simulink model "model_FS_PSH_IEEE39"  (R2020b)
settings: Solver=ode3  StartTime=0.0  StopTime=300  FixedStep=Ts  RelTol=1e-3
PostLoadFcn:
  | IEEE39BusLineLength;
  | vNomHV = 345E3;fNom=60;load('Dynamicload.mat');
InitFcn:
  | IEEE39BusLineLength;
  | vNomHV = 345E3;fNom=60;load('Dynamicload.mat');
values from neighbouring files (symbols this model uses):
  Rp = 0.05    [IEEE39BusLineLength.m]
  t_sw_off = 220    [MAIN_FS_PSH_IEEE39.m]    (also in MAIN_T_PSH_IEEE39.m; MAIN_VS_PSH.m = 45)
  t_sw_on = 130    [MAIN_FS_PSH_IEEE39.m]    (also in MAIN_T_PSH_IEEE39.m; MAIN_VS_PSH.m = 35)
  TL_10_11_len = 14    [IEEE39BusLineLength.m]
  TL_10_13_len = 14    [IEEE39BusLineLength.m]
  TL_13_14_len = 32    [IEEE39BusLineLength.m]
  TL_14_15_len = 70    [IEEE39BusLineLength.m]
  TL_15_16_len = 31.5    [IEEE39BusLineLength.m]
  TL_16_17_len = 26    [IEEE39BusLineLength.m]
  TL_16_19_len = 61    [IEEE39BusLineLength.m]
  TL_16_21_len = 46    [IEEE39BusLineLength.m]
  TL_16_24_len = 15    [IEEE39BusLineLength.m]
  TL_17_18_len = 26    [IEEE39BusLineLength.m]
  TL_17_27_len = 59    [IEEE39BusLineLength.m]
  TL_1_2_len = 134    [IEEE39BusLineLength.m]
  TL_1_39_len = 105    [IEEE39BusLineLength.m]
  TL_21_22_len = 47    [IEEE39BusLineLength.m]
  TL_22_23_len = 33    [IEEE39BusLineLength.m]
  TL_24_23_len = 88    [IEEE39BusLineLength.m]
  TL_25_26_len = 101    [IEEE39BusLineLength.m]
  TL_26_27_len = 46.5    [IEEE39BusLineLength.m]
  TL_26_28_len = 151    [IEEE39BusLineLength.m]
  TL_26_29_len = 200    [IEEE39BusLineLength.m]
  TL_28_29_len = 48    [IEEE39BusLineLength.m]
  TL_2_25_len = 28    [IEEE39BusLineLength.m]
  TL_2_2_len = 49    [IEEE39BusLineLength.m]
  TL_3_18_len = 42    [IEEE39BusLineLength.m]
  TL_3_4_len = 53    [IEEE39BusLineLength.m]
  TL_4_14_len = 33    [IEEE39BusLineLength.m]
  TL_4_5_len = 32.5    [IEEE39BusLineLength.m]
  TL_5_6_len = 14    [IEEE39BusLineLength.m]
  TL_5_8_len = 32    [IEEE39BusLineLength.m]
  TL_6_11_len = 26.5    [IEEE39BusLineLength.m]
  TL_6_7_len = 25.5    [IEEE39BusLineLength.m]
  TL_7_8_len = 15    [IEEE39BusLineLength.m]
  TL_8_9_len = 93    [IEEE39BusLineLength.m]
  TL_9_39_len = 136    [IEEE39BusLineLength.m]
  Ts = 25e-6    (= 2.5e-05)    [MAIN_FS_PSH_IEEE39.m]    (also in MAIN_T_PSH_IEEE39.m; MAIN_VS_PSH.m = 1e-07)
undefined symbols (not defined in the file or in its folder): D1, Delta, FS_PSH, load15, load16, load18, load20, load21, load23, load24, load25, load26, load27, load28, load29, load3, load39, load4, load7, load8
libraries: powerlib x216, sps_avr x10, powerlib_meascontrol x5, pid_lib x1
(part 1 of 8)
settings Model: ARTEMISmethode_block_infos=$$__separator__$$IEEE39bus_60Hz/ARTEMIS Guide$$__separator__$$  SimulationMode=accelerator  Creator=Admin  LastModifiedBy=mjimene
settings DataIOCC: LimitDataPoints=on  SaveFormat=Array  SignalLoggingSaveFormat=ModelDataLogs  SaveOutput=off  SignalLogging=off  DSMLogging=off  SaveTime=off
settings OptimizationCC: BlockReduction=off  OptimizeBlockIOStorage=off  BufferReuse=off  GlobalBufferReuse=off  ExpressionFolding=off  ExpressionDepthLimit=2147483647  LocalBlockOutputs=off  LifeSpan=inf
settings DebuggingCC: UnderspecifiedInitializationDetection=Classic  MergeDetectMultiDrivingBlocksExec=none  SolverPrmCheckMsg=warning  FcnCallInpInsideContextMsg=warning  UnconnectedInputMsg=none  UnconnectedOutputMsg=none  UnconnectedLineMsg=none  StateNameClashWarn=warning  SFUnexpectedBacktrackingDiag=warning  SFNoUnconditionalDefaultTransitionDiag=warning  SFExecutionAtInitializationDiag=none  ArithmeticOperatorsInVariantConditions=warning
settings HardwareCC: ProdBitPerPointer=32  ProdBitPerSizeT=32  ProdBitPerPtrDiffT=32  ProdLargestAtomicFloat=None  ProdIntDivRoundTo=Undefined  ProdEndianess=Unspecified  ProdWordSize=32  ProdHWDeviceType=32-bit Generic
settings ModelReferenceCC: PropagateSignalLabelsOutOfModel=off
settings SFSimCC: SimUseLocalCustomCode=off  CustomCodeUndefinedFunction=UseInterfaceOnly
settings RTWCC: RTWUseLocalCustomCode=off
settings CodeAppCC: StateflowObjectComments=on
settings GRTTargetCC: TargetLangStandard=C89/C90 (ANSI)  CombineOutputUpdateFcns=off  GRTInterface=on
settings ConfigComp: CovMetricSettings=dw  CovSaveCumulativeToWorkspaceVar=on  CovSaveSingleToWorkspaceVar=on  CovExternalEMLEnable=off
settings SimscapeCC: SimscapeNormalizeSystem=off

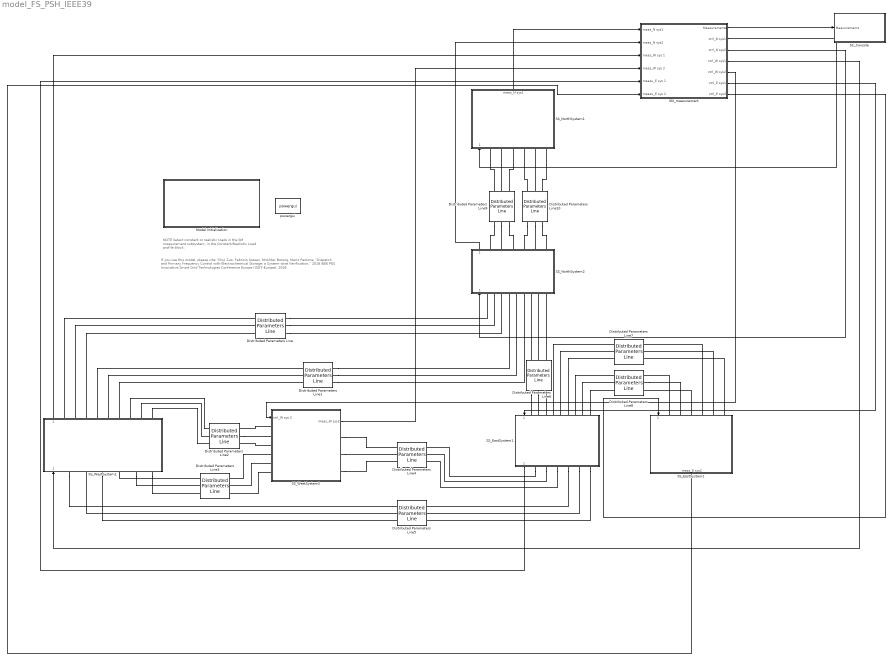
== system model_FS_PSH_IEEE39 ==
  note: If you use this model, please cite:
      | Yihui Zuo, Fabrizio Sossan, Mokhtar Bozorg, Mario Paolone,
      | “Dispatch and Primary Frequency Control with Electrochemical Storage: a System-wise Verification,”
      | 2018 IEEE PES Innovative Smart Grid Technologies Conference Europe (ISGT-Europe), 2018.
  note: NOTE
      | Select constant or realistic loads in the SM measurement
      | subsystem, in the Constant/Realistic Load profile block.
  Distributed Parameters Line : powerlib/Elements/Distributed Parameters Line  Phases=3  Length=TL_1_39_len  Frequency=fNom  Resistance=[1.19 4.76]/TL_1_39_len  Inductance="[0.079  0.237]/TL_1_39_len"  Capacitance=[1.67e-6 0.7599e-6]/TL_1_39_len  x1=[-0.000425 4.88875301437083e-09 0 0;-0.0004 4.8690649712249e-09 0 0;-0.000375 4.84894442957481e-09 175040.631407091 -214779.963387365;-0.00035 4.8283931766434e-09 177057.068450198 -213120.729509055;-0.000325 4.80741303791179e-09 179057.778260723 -211442.565015264;-0.0003 4.7860058769572e-09 181042.583124052 -209745.618970267;-0.000275 4.76417359528746e-09 183011.306738343 -208030.042106622;-0.00025 4.74191813217205e-09 184963.774230179 -206295.986811787;-0.000225 4.7192414644699e-09 186899.812170109 -204543.607114579;-0.0002 4.69614560645374e-09 188819.248588048 -202773.058671495;-0.000175 4.67263260963124e-09 190721.912988556 -200984.498752886;-0.00015 4.64870456256271e-09 192607.636365979 -199178.086228986;-0.000125 4.62436359067567e-09 194476.251219464 -197353.981555798;-0.0001 4.59961185607596e-09 196327.591567834 -195512.346760849;-7.5e-05 4.57445155735578e-09 198161.492964335 -193653.345428788;-5e-05 4.54888492939834e-09 199977.792511241 -191777.142686863;-2.5e-05 4.52291424317936e-09 201776.328874325 -189883.90519025]  x2=[-0.000425 -1.83196451090801e-09 0 0;-0.0004 -1.83078345578025e-09 0 0;-0.000375 -1.82943977988018e-09 182487.482258839 -212730.350697277;-0.00035 -1.82793360256085e-09 184484.271802376 -211001.024061735;-0.000325 -1.82626505760965e-09 186464.674386185 -209252.955095208;-0.0003 -1.82443429323639e-09 188428.514099458 -207486.299071287;-0.000275 -1.82244147206013e-09 190375.616502595 -205701.212914576;-0.00025 -1.82028677109479e-09 192305.808642704 -203897.855186749;-0.000225 -1.81797038173336e-09 194218.919068958 -202076.386072467;-0.0002 -1.81549250973094e-09 196114.777847827 -200236.967365147;-0.000175 -1.81285337518644e-09 197993.216578172 -198379.762452596;-0.00015 -1.81005321252306e-09 199854.068406204 -196504.936302493;-0.000125 -1.80709227046743e-09 201697.168040304 -194612.655447735;-0.0001 -1.80397081202756e-09 203522.351765705 -192703.087971651;-7.5e-05 -1.80068911446941e-09 205329.457459036 -190776.403493065;-5e-05 -1.79724746929236e-09 207118.324602719 -188832.773151232;-2.5e-05 -1.79364618220321e-09 208888.794299233 -186872.369590637]  x3=[-0.000425 -1.8959273665696e-11 0 0;-0.0004 -1.96784433016388e-11 0 0;-0.000375 -2.03958649844648e-11 812.638231026358 -1285.4974921655;-0.00035 -2.11114749886319e-11 824.717434819385 -1277.78157783389;-0.000325 -2.18252097495219e-11 836.723382441253 -1269.95216355427;-0.0003 -2.25370058690864e-11 848.655007454274 -1262.0099447805;-0.000275 -2.32468001214783e-11 860.511250022524 -1253.95562698636;-0.00025 -2.39545294586682e-11 872.291057005985 -1245.78992560294;-0.000225 -2.4660131016044e-11 883.993382054088 -1237.51356595505;-0.0002 -2.53635421179956e-11 895.617185698659 -1229.1272831968;-0.000175 -2.60647002834817e-11 907.161435446248 -1220.63182224631;-0.00015 -2.676354323158e-11 918.625105869841 -1212.02793771956;-0.000125 -2.74600088870189e-11 930.007178699949 -1203.31639386332;-0.0001 -2.8154035385692e-11 941.306642915049 -1194.49796448727;-7.5e-05 -2.88455610801526e-11 952.522494831397 -1185.57343289531;-5e-05 -2.95345245450902e-11 963.653738192173 -1176.54359181594;-2.5e-05 -3.02208645827861e-11 974.69938425598 -1167.40924333185]  x4=[-0.000425 2.59415673625815e-11 0 0;-0.0004 2.66310740131385e-11 0 0;-0.000375 2.73182151377182e-11 690.026985476241 -784.438717599278;-0.00035 2.80029297004726e-11 697.389331159264 -777.900629917322;-0.000325 2.86851568810953e-11 704.689730689518 -771.293444603517;-0.0003 2.93648360802234e-11 711.927535603305 -764.617748546266;-0.000275 3.00419069248204e-11 719.102102996943 -757.874134719492;-0.00025 3.0716309273539e-11 726.212795583873 -751.063202129969;-0.000225 3.13879832220632e-11 733.258981751264 -744.185555764109;-0.0002 3.20568691084291e-11 740.240035616118 -737.241806534231;-0.000175 3.27229075183247e-11 747.155337080867 -730.23257122429;-0.00015 3.33860392903674e-11 754.004271888449 -723.158472435095;-0.000125 3.4046205521359e-11 760.786231676874 -716.020138529004;-0.0001 3.47033475715175e-11 767.500614033259 -708.818203574108;-7.5e-05 3.53574070696866e-11 774.146822547339 -701.553307287913;-5e-05 3.60083259185195e-11 780.724266864447 -694.226094980512;-2.5e-05 3.66560462996407e-11 787.232362737945 -686.837217497271]  x5=0.000424377544174995  V1=ones(3,3)  V2=ones(3,3)  I1=ones(3,3)  I2=ones(3,3)  nHarmo=1  Measurements=None  Decoupling=off  VsMag0=0  VrMag0=0  VsAngle0=0  VrAngle0=0  IsMag0=0  IrMag0=0  IsAngle0=0  IrAngle0=0
  Distributed Parameters Line1 : powerlib/Elements/Distributed Parameters Line  Phases=3  Length=TL_3_4_len  Frequency=fNom  Resistance=[1.547 6.18]/TL_3_4_len  Inductance="[0.067  0.208]/TL_3_4_len"  Capacitance=[0.493e-6 0.224e-6]/TL_3_4_len  x1=[-0.000225 1.5632362654316e-09 0 0;-0.0002 1.38665566248243e-09 164719.624177691 -206950.281139344;-0.000175 1.20995188875953e-09 166662.729017853 -205388.66612348;-0.00015 1.0331406401138e-09 168591.029910762 -203808.807298714;-0.000125 8.56237621942703e-10 170504.355573585 -202210.84499724;-0.0001 6.79258547795169e-10 172402.536053672 -200594.92115931;-7.5e-05 5.02219137975879e-10 174285.402743659 -198961.179320623;-5e-05 3.25135118148872e-10 176152.788396437 -197309.764599575;-2.5e-05 1.48022217940708e-10 178004.527140018 -195640.823684371]  x2=[-0.000225 8.25262885618808e-10 0 0;-0.0002 7.17563772164822e-10 180495.051613948 -202247.997497279;-0.000175 6.09800920547568e-10 182393.138299879 -200537.913661572;-0.00015 5.0198390288662e-10 184275.023772651 -198810.016888842;-0.000125 3.94122296112896e-10 186140.540872315 -197064.460660873;-0.0001 2.86225681117977e-10 187989.523892855 -195301.400028062;-7.5e-05 1.78303641903076e-10 189821.808596909 -193520.991595647;-5e-05 7.03657647277308e-11 191637.232230355 -191723.393509802;-2.5e-05 -3.75783627416992e-11 193435.633536768 -189908.765443581]  x3=[-0.000225 -9.04367168497082e-11 0 0;-0.0002 -9.06321895354064e-11 649.467044553634 -1184.96845355775;-0.000175 -9.08196117459856e-11 660.606070103996 -1178.79484024844;-0.00015 -9.09989668335215e-11 671.686416803521 -1172.51651956552;-0.000125 -9.1170238866658e-11 682.707100431747 -1166.13404918572;-0.0001 -9.13334126320229e-11 693.667142067832 -1159.64799603696;-7.5e-05 -9.14884736355789e-11 704.565568177505 -1153.058936248;-5e-05 -9.16354081039111e-11 715.401410699543 -1146.36745509721;-2.5e-05 -9.17742029854503e-11 726.173707131761 -1139.57414696065]  x4=[-0.000225 9.50905553689282e-11 0 0;-0.0002 9.49819209215151e-11 246.058671175114 46.4396508064798;-0.000175 9.48648496306908e-11 245.610034551809 48.7566113817653;-0.00015 9.47393518954042e-11 245.139581425092 51.0692411129122;-0.000125 9.46054388630899e-11 244.647353583332 53.3773345787761;-0.0001 9.44631224286775e-11 244.133394749051 55.6806867611495;-7.5e-05 9.43124152335358e-11 243.597750575044 57.9790930629735;-5e-05 9.41533306643492e-11 243.040468640325 60.2723493265106;-2.5e-05 9.3985882851929e-11 242.461598445897 62.5602518514799]  x5=0.000215851801011713  V1=ones(3,3)  V2=ones(3,3)  I1=ones(3,3)  I2=ones(3,3)  nHarmo=1  Measurements=None  Decoupling=off  VsMag0=0  VrMag0=0  VsAngle0=0  VrAngle0=0  IsMag0=0  IrMag0=0  IsAngle0=0  IrAngle0=0
  Distributed Parameters Line10 : powerlib/Elements/Distributed Parameters Line  Phases=3  Length=TL_2_25_len  Frequency=fNom  Resistance=[8.33 33.3]/TL_2_25_len  Inductance=[0.027 0.082]/TL_2_25_len  Capacitance=[0.325e-6 0.148e-6]/TL_2_25_len  x1=[-0.000125 -1.52411133679905e-08 0 0;-0.0001 -1.52689723349653e-08 209999.096747657 -182360.400508997;-7.5e-05 -1.52954750235306e-08 211708.439215037 -180373.134567961;-5e-05 -1.53206190795644e-08 213398.976514727 -178369.846842178;-2.5e-05 -1.53444022696261e-08 215070.558483429 -176350.715275245]  x2=[-0.000125 -3.23132321557523e-09 0 0;-0.0001 -3.46465111979732e-09 215023.64160142 -177308.507218749;-7.5e-05 -3.697671273674e-09 216685.148783807 -175274.111353792;-5e-05 -3.93036297900783e-09 218327.408738383 -173224.146628811;-2.5e-05 -4.16270556677612e-09 219950.275590124 -171158.795133528]  x3=[-0.000125 4.89699895493984e-10 0 0;-0.0001 4.88043403374434e-10 1233.51381638052 -683.564878713321;-7.5e-05 4.86343560417879e-10 1239.90136407071 -671.909097165952;-5e-05 4.84600517614202e-10 1246.1787765525 -660.193632767527;-2.5e-05 4.8281442979054e-10 1252.34549622983 -648.419526153335]  x4=[-0.000125 -5.06467605037126e-10 0 0;-0.0001 -5.05184942665193e-10 187.77424541273 -563.224558463668;-7.5e-05 -5.03857406845621e-10 193.074034709732 -561.429834212542;-5e-05 -5.0248511549782e-10 198.356674054597 -559.585240517297;-2.5e-05 -5.01068190516641e-10 203.621694212755 -557.690941225411]  x5=0.000110163514831363  V1=ones(3,3)  V2=ones(3,3)  I1=ones(3,3)  I2=ones(3,3)  nHarmo=1  Measurements=None  Decoupling=off  VsMag0=0  VrMag0=0  VsAngle0=0  VrAngle0=0  IsMag0=0  IrMag0=0  IsAngle0=0  IrAngle0=0
  Distributed Parameters Line2 : powerlib/Elements/Distributed Parameters Line  Phases=3  Length=TL_5_6_len  Frequency=fNom  Resistance=[0.476 1.904]/TL_5_6_len  Inductance=[0.014 0.04]/TL_5_6_len  Capacitance=[0.162e-6 0.074e-6]/TL_5_6_len  x1=[-7.5e-05 5.17945332679916e-09 0 0;-5e-05 5.02501749446172e-09 181587.362366807 -193505.62103115;-2.5e-05 4.87013531101526e-09 183403.006839299 -191785.629766195]  x2=[-7.5e-05 4.57233624476333e-09 0 0;-5e-05 4.4067894411438e-09 186742.152897159 -190041.198023314;-2.5e-05 4.24085120100561e-09 188524.917480904 -188272.778460778]  x3=[-7.5e-05 7.52806130754931e-11 0 0;-5e-05 7.46047227504442e-11 1348.9677163105 -1572.38235268503;-2.5e-05 7.39222056025487e-11 1363.72687786416 -1559.59898034527]  x4=[-7.5e-05 -6.46675614638656e-11 0 0;-5e-05 -6.44345072798196e-11 -109.2519168985 258.023491005601;-2.5e-05 -6.41957296502703e-11 -111.678857189618 256.982378873185]  x5=5.44058820349418e-05  V1=ones(3,3)  V2=ones(3,3)  I1=ones(3,3)  I2=ones(3,3)  nHarmo=1  Measurements=None  Decoupling=off  VsMag0=0  VrMag0=0  VsAngle0=0  VrAngle0=0  IsMag0=0  IrMag0=0  IsAngle0=0  IrAngle0=0
  Distributed Parameters Line3 : powerlib/Elements/Distributed Parameters Line  Phases=3  Length=TL_7_8_len  Frequency=fNom  Resistance=[0.476 1.904]/TL_7_8_len  Inductance=[0.015 0.044]/TL_7_8_len  Capacitance=[0.174e-6 0.079e-6]/TL_7_8_len  x1=[-7.5e-05 5.70090851640329e-09 171457.428300872 -200312.665773904;-5e-05 5.542472475404e-09 173337.67644286 -198687.843222525;-2.5e-05 5.38354411995231e-09 175202.52773017 -197045.372068077]  x2=[-7.5e-05 3.96483863419745e-09 173653.247691791 -198600.78990211;-5e-05 3.80286132220067e-09 175517.264541132 -196955.34854543;-2.5e-05 3.64054621807272e-09 177365.690932178 -195292.412475876]  x3=[-7.5e-05 1.62209346020676e-11 909.488322420405 -1047.03494594747;-5e-05 1.49784533403536e-11 919.315811611816 -1038.41683200806;-2.5e-05 1.37346416058071e-11 929.061641857264 -1029.7064798814]  x4=[-7.5e-05 -9.64506437720554e-12 251.4146560831 -321.274619857994;-5e-05 -8.89088497789997e-12 254.431353309077 -318.890860654254;-2.5e-05 -8.13591583878269e-12 257.425450471106 -316.478775720412]  x5=5.89576118919347e-05  V1=ones(3,3)  V2=ones(3,3)  I1=ones(3,3)  I2=ones(3,3)  nHarmo=1  Measurements=None  Decoupling=off  VsMag0=0  VrMag0=0  VsAngle0=0  VrAngle0=0  IsMag0=0  IrMag0=0  IsAngle0=0  IrAngle0=0
  Distributed Parameters Line4 : powerlib/Elements/Distributed Parameters Line  Phases=3  Length=TL_13_14_len  Frequency=fNom  Resistance=[1.071 4.285]/TL_13_14_len  Inductance=[0.032 0.095]/TL_13_14_len  Capacitance=[0.384e-6 0.175e-6]/TL_13_14_len  x1=[-0.00015 -1.81496385128925e-08 0 0;-0.000125 -1.82986977397538e-08 185893.773668375 -192778.554928865;-0.0001 -1.84461315704769e-08 187702.375329091 -191018.011094471;-7.5e-05 -1.85919269091365e-08 189494.304179516 -189240.499935845;-5e-05 -1.87360708053477e-08 191269.401050169 -187446.179341807;-2.5e-05 -1.88785504554162e-08 193027.508266682 -185635.208694288]  x2=[-0.00015 -3.52435583854237e-10 0 0;-0.000125 -5.14562608948772e-10 176946.023237204 -199124.857360815;-0.0001 -6.76643927617127e-10 178814.833709439 -197448.360585469;-7.5e-05 -8.38665142859408e-10 180667.760814219 -195754.32530507;-5e-05 -1.00061186301445e-09 182504.639963845 -194042.901993626;-2.5e-05 -1.16246970303819e-09 184325.307996088 -192314.242669652]  x3=[-0.00015 7.12349736466559e-11 0 0;-0.000125 7.55672293907323e-11 41.8929000513877 9.12609117373639;-0.0001 7.98927728165569e-11 41.8049593803182 9.52049914718043;-7.5e-05 8.42112197043519e-11 41.713305351036 9.91406145484175;-5e-05 8.8522186464695e-11 41.6179461047821 10.3067431382405;-2.5e-05 9.28252901725922e-11 41.518890111916 10.6985093171192]  x4=[-0.00015 -9.39950019429511e-11 0 0;-0.000125 -9.87567150264296e-11 1183.21024928078 -1389.16538870043;-0.0001 -1.03509655967458e-10 1196.25007813283 -1377.95234845843;-7.5e-05 -1.08253402582341e-10 1209.18364913609 -1366.61691052139;-5e-05 -1.12987533504073e-10 1222.00981345602 -1355.16008176843;-2.5e-05 -1.17711628219775e-10 1234.72743179853 -1343.58287986135]  x5=0.000128937969582276  V1=ones(3,3)  V2=ones(3,3)  I1=ones(3,3)  I2=ones(3,3)  nHarmo=1  Measurements=None  Decoupling=off  VsMag0=0  VrMag0=0  VsAngle0=0  VrAngle0=0  IsMag0=0  IrMag0=0  IsAngle0=0  IrAngle0=0
  Distributed Parameters Line5 : powerlib/Elements/Distributed Parameters Line  Phases=3  Length=TL_4_14_len  Frequency=fNom  Resistance=[0.9522 3.808]/TL_4_14_len  Inductance=[0.041 0.1223]/TL_4_14_len  Capacitance=[0.308e-6 0.14e-6]/TL_4_14_len  x1=[-0.00015 1.0331406401138e-09 0 0;-0.000125 8.56237621942703e-10 170504.355573585 -202210.84499724;-0.0001 6.79258547795169e-10 172402.536053672 -200594.92115931;-7.5e-05 5.02219137975879e-10 174285.402743659 -198961.179320623;-5e-05 3.25135118148872e-10 176152.788396437 -197309.764599575;-2.5e-05 1.48022217940708e-10 178004.527140018 -195640.823684371]  x2=[-0.00015 -3.52435583854237e-10 0 0;-0.000125 -5.14562608948772e-10 176946.023237204 -199124.857360815;-0.0001 -6.76643927617127e-10 178814.833709439 -197448.360585469;-7.5e-05 -8.38665142859408e-10 180667.760814219 -195754.32530507;-5e-05 -1.00061186301445e-09 182504.639963845 -194042.901993626;-2.5e-05 -1.16246970303819e-09 184325.307996088 -192314.242669652]  x3=[-0.00015 -3.42245806602751e-11 0 0;-0.000125 -3.46643607029233e-11 678.924113850406 -965.55701602572;-0.0001 -3.51010616566211e-11 687.993983330425 -959.115491615321;-7.5e-05 -3.55346447310646e-11 697.002741206795 -952.588773021254;-5e-05 -3.59650714128982e-11 705.949587269551 -945.977439984403;-2.5e-05 -3.63923034691353e-11 714.833726808094 -939.282079761596]  x4=[-0.00015 3.59920205374366e-11 0 0;-0.000125 3.60665207540646e-11 248.24579667473 -152.436724387801;-0.0001 3.6137817333779e-11 249.671376317893 -150.09035023835;-7.5e-05 3.62059039436053e-11 251.074778705787 -147.730644196153;-5e-05 3.62707745356972e-11 252.455879180096 -145.357815863946;-2.5e-05 3.63324233478735e-11 253.814555063491 -142.97207601006]  x5=0.000130851060370178  V1=ones(3,3)  V2=ones(3,3)  I1=ones(3,3)  I2=ones(3,3)  nHarmo=1  Measurements=None  Decoupling=off  VsMag0=0  VrMag0=0  VsAngle0=0  VrAngle0=0  IsMag0=0  IrMag0=0  IsAngle0=0  IrAngle0=0
  Distributed Parameters Line6 : powerlib/Elements/Distributed Parameters Line  Phases=3  Length=TL_16_17_len  Frequency=fNom  Resistance=[0.8332 3.33]/TL_16_17_len  Inductance=[0.028 0.084]/TL_16_17_len  Capacitance=[0.299e-6 0.136e-6]/TL_16_17_len  x1=[-0.000125 3.4902500343367e-08 0 0;-0.0001 3.46336269469464e-08 176282.624522429 -204235.907809339;-7.5e-05 3.43616771915251e-08 178199.634824584 -202565.435936314;-5e-05 3.40866752332531e-08 180100.816404805 -200876.971030016;-2.5e-05 3.38086454993943e-08 181986.000389152 -199170.66306966]  x2=[-0.000125 2.16125954865691e-08 0 0;-0.0001 2.13654534678538e-08 179085.783169739 -203138.687259504;-7.5e-05 2.11164136460244e-08 180992.327499674 -201441.845312146;-5e-05 2.08654981422377e-08 182882.795044564 -199727.110135331;-2.5e-05 2.06127292442597e-08 184757.017882151 -197994.634041752]  x3=[-0.000125 -6.7563457940461e-11 0 0;-0.0001 -7.16937803309209e-11 687.376123293795 -931.430025702937;-7.5e-05 -7.58177344652712e-11 696.123944500083 -924.910436669318;-5e-05 -7.99349540300604e-11 704.809931952561 -918.308691742789;-2.5e-05 -8.40450733100409e-11 713.433314111602 -911.625377328507]  x4=[-0.000125 1.41228119556839e-10 0 0;-0.0001 1.44745416475713e-10 448.600176002786 -417.079838335438;-7.5e-05 1.48249856269763e-10 452.511053073745 -412.833363648834;-5e-05 1.51741127654384e-10 456.381735496506 -408.550218715827;-2.5e-05 1.55218920514664e-10 460.211879454675 -404.230783990115]  x5=0.000106883113727099  V1=ones(3,3)  V2=ones(3,3)  I1=ones(3,3)  I2=ones(3,3)  nHarmo=1  Measurements=None  Decoupling=off  VsMag0=0  VrMag0=0  VsAngle0=0  VrAngle0=0  IsMag0=0  IrMag0=0  IsAngle0=0  IrAngle0=0
  Distributed Parameters Line7 : powerlib/Elements/Distributed Parameters Line  Phases=3  Length=TL_16_21_len  Frequency=fNom  Resistance=[0.9522 3.809]/TL_16_21_len  Inductance=[0.043 0.128]/TL_16_21_len  Capacitance=[0.568e-6 0.258e-6]/TL_16_21_len  x1=[-0.0002 3.56904249287326e-08 0 0;-0.000175 3.54309228030293e-08 170438.331022878 -209137.88948923;-0.00015 3.51682734978974e-08 172401.800262951 -207522.280543111;-0.000125 3.4902500343367e-08 174349.955778281 -205888.23826812;-0.0001 3.46336269469464e-08 176282.624522429 -204235.907809339;-7.5e-05 3.43616771915251e-08 178199.634824584 -202565.435936314;-5e-05 3.40866752332531e-08 180100.816404805 -200876.971030016;-2.5e-05 3.38086454993943e-08 181986.000389152 -199170.66306966]  x2=[-0.0002 1.55933291358479e-08 0 0;-0.000175 1.53513573320371e-08 176314.466791581 -201742.801147765;-0.00015 1.51080219319049e-08 178207.978996054 -200072.140420211;-0.000125 1.48633445499086e-08 180085.661737416 -198383.708128307;-0.0001 1.46173469197081e-08 181947.348229028 -196677.654248373;-7.5e-05 1.43700508922352e-08 183792.873105134 -194954.130321979;-5e-05 1.41214784337529e-08 185622.072435541 -193213.289442485;-2.5e-05 1.38716516239044e-08 187434.783740189 -191455.286241445]  x3=[-0.0002 -1.71998150069946e-11 0 0;-0.000175 -2.14012866166488e-11 1070.76302096095 -1110.52463854068;-0.00015 -2.56008572402814e-11 1081.1817362093 -1100.38376291479;-0.000125 -2.97981538477471e-11 1091.50441464435 -1090.14514484055;-0.0001 -3.39928036108922e-11 1101.73013934609 -1079.80969377122;-7.5e-05 -3.81844339366707e-11 1111.85800200655 -1069.37832776132;-5e-05 -4.23726725002408e-11 1121.88710301039 -1058.85197338509;-2.5e-05 -4.65571472780363e-11 1131.81655151488 -1048.2315656542]  x4=[-0.0002 9.11251245888991e-11 0 0;-0.000175 9.46578323409228e-11 142.301427146099 -416.005218226123;-0.00015 9.81821320369568e-11 146.215754731806 -414.645599045362;-0.000125 1.01697710628324e-10 150.117094588743 -413.249148644971;-0.0001 1.05204255841008e-10 154.005100177346 -411.815991065749;-7.5e-05 1.08701456203386e-10 157.879426142479 -410.34625360904;-5e-05 1.12189001073901e-10 161.739728344108 -408.840066825422;-2.5e-05 1.15666580668652e-10 165.585663887869 -407.297564503114]  x5=0.000181725067065609  V1=ones(3,3)  V2=ones(3,3)  I1=ones(3,3)  I2=ones(3,3)  nHarmo=1  Measurements=None  Decoupling=off  VsMag0=0  VrMag0=0  VsAngle0=0  VrAngle0=0  IsMag0=0  IrMag0=0  IsAngle0=0  IrAngle0=0
  Distributed Parameters Line8 : powerlib/Elements/Distributed Parameters Line  Phases=3  Length=TL_16_24_len  Frequency=fNom  Resistance=[0.357 1.428]/TL_16_24_len  Inductance=[0.019 0.056]/TL_16_24_len  Capacitance=[0.152e-6 0.069e-6]/TL_16_24_len  x1=[-7.5e-05 3.43616771915251e-08 178199.634824584 -202565.435936314;-5e-05 3.40866752332531e-08 180100.816404805 -200876.971030016;-2.5e-05 3.38086454993943e-08 181986.000389152 -199170.66306966]  x2=[-7.5e-05 3.17888723853282e-08 178605.931508548 -204519.772572357;-5e-05 3.1546638855704e-08 180525.513946055 -202827.391761394;-2.5e-05 3.13016031712108e-08 182429.061063597 -201116.994648726]  x3=[-7.5e-05 -1.36689940585158e-10 228.611592167635 -647.725370705071;-5e-05 -1.38016526015978e-10 234.70600061128 -645.542021070987;-2.5e-05 -1.39330852020932e-10 240.779561110859 -643.301330662002]  x4=[-7.5e-05 2.08134738064355e-10 768.164986587064 -513.031984667701;-5e-05 2.08892675568913e-10 772.965969870192 -505.769516559255;-2.5e-05 2.09632058018189e-10 777.698293846509 -498.462123077939]  x5=6.21610810716802e-05  V1=ones(3,3)  V2=ones(3,3)  I1=ones(3,3)  I2=ones(3,3)  nHarmo=1  Measurements=None  Decoupling=off  VsMag0=0  VrMag0=0  VsAngle0=0  VrAngle0=0  IsMag0=0  IrMag0=0  IsAngle0=0  IrAngle0=0
  Distributed Parameters Line9 : powerlib/Elements/Distributed Parameters Line  Phases=3  Length=TL_26_27_len  Frequency=fNom  Resistance=[1.666 6.665]/TL_26_27_len  Inductance=[0.046 0.139]/TL_26_27_len  Capacitance=[0.534e-6 0.243e-6]/TL_26_27_len  x1=[-0.0002 1.21376014343686e-08 0 0;-0.000175 1.18590072463739e-08 175488.272737464 -207699.435035008;-0.00015 1.15793596727857e-08 177437.959643062 -206036.296011196;-0.000125 1.12986835535183e-08 179371.88548312 -204354.855652249;-0.0001 1.10170038198476e-08 181289.878475163 -202655.263313423;-7.5e-05 1.07343454921961e-08 183191.768251964 -200937.669962337;-5e-05 1.0450733677911e-08 185077.385876676 -199202.228165563;-2.5e-05 1.01661935690334e-08 186946.563857838 -197449.092075075]  x2=[-0.0002 7.87032423702723e-09 0 0;-0.000175 7.56171786436313e-09 189804.535214744 -200237.563954282;-0.00015 7.2524398161957e-09 191683.260425392 -198439.830698471;-0.000125 6.94251756438947e-09 193544.959220518 -196624.470869499;-0.0001 6.63197863803083e-09 195389.466233269 -194791.645718121;-7.5e-05 6.3208506209828e-09 197216.617623868 -192941.518046466;-5e-05 6.00916114943481e-09 199026.251094163 -191074.25219357;-2.5e-05 5.69693790944797e-09 200818.205902046 -189190.014020785]  x3=[-0.0002 6.65401004961945e-11 0 0;-0.000175 6.53446365348635e-11 1078.27020274046 -1497.59705814019;-0.00015 6.41433682850862e-11 1092.33658172448 -1487.3682609482;-0.000125 6.29364024504544e-11 1106.3059330573 -1477.00734710716;-0.0001 6.17238462406523e-11 1120.17701590038 -1466.51523693334;-7.5e-05 6.05058073619337e-11 1133.94859814393 -1455.89286239664;-5e-05 5.92823940075546e-11 1147.61945651639 -1445.14116703779;-2.5e-05 5.8053714848163e-11 1161.18837669308 -1434.26110588452]  x4=[-0.0002 -3.79813109267231e-11 0 0;-0.000175 -3.75594274698902e-11 120.094014769625 76.9223216081484;-0.00015 -3.7134207767537e-11 119.363680821452 78.0507745719642;-0.000125 -3.67056895901362e-11 118.622744300975 79.1722946146852;-0.0001 -3.627391100115e-11 117.871271022462 80.2867821164164;-7.5e-05 -3.58389103536493e-11 117.109327736112 81.3941380819337;-5e-05 -3.54007262869068e-11 116.336982122135 82.4942641494775;-2.5e-05 -3.4959397722965e-11 115.554302784734 83.5870625994895]  x5=0.000183785200709959  V1=ones(3,3)  V2=ones(3,3)  I1=ones(3,3)  I2=ones(3,3)  nHarmo=1  Measurements=None  Decoupling=off  VsMag0=0  VrMag0=0  VsAngle0=0  VrAngle0=0  IsMag0=0  IrMag0=0  IsAngle0=0  IrAngle0=0
  Model Initialization : Subsystem  AncestorBlock=artemis/Tools /Misc/Model Initialization  mask(Model Functions){InitFcnX=|, prel=off, posl=on, inif=on, strf=off}
      mask InitFcnX=|
      | IEEE39BusLineLength;
      | vNomHV = 345E3;fNom=60;load('Dynamicload.mat');
      mask prompts: InitFcnX "Initialisation"; prel "Preload Function"; posl "PostLoad Function"; inif "InitFcn"; strf "StartFcn"
      mask init:
      | currentBlock = gcb;
      | root = bdroot(currentBlock);
      | 
      | if ~strcmp(get_param(root,'BlockDiagramType'),'library')
      |     if prel==1
      |         set_param(root, 'PreLoadFcn', InitFcnX);
      |     else
      |         set_param(root, 'PreLoadFcn', '');
      |     end
      |     if inif==1
      |         set_param(root, 'InitFcn', InitFcnX);
      |     else
      |         set_param(root, 'InitFcn', '');
      |     end
      |     if strf==1
      |         set_param(root, 'StartFcn', InitFcnX);
      |     else
      |         set_param(root, 'StartFcn', '');
      |     end
      |     if posl==1
      |         set_param(root, 'PostLoadFcn', InitFcnX);
      |     else
      |         set_param(root, 'PostLoadFcn', '');
      |     end
      | end
      | 
      | pos = get_param(currentBlock, 'Position');
      | width = pos(3) - pos(1); height = pos(4) - pos(2);
      | txt = [ upper(root) '\n' '- InitFcn. . . . . '  get_param(root, 'InitFcn') ];
      settings: CopyFcn=set_param(gcb,'LinkStatus','inactive')
      mask Display: text(5, height*0.5, txt, 'horizontalAlignment', 'left', 'verticalAlignment', 'middle') ;
  SC_Console : Subsystem
  SM_measurement : Subsystem
  SS_EastSystem1 : Subsystem
      mask Display: disp('Eastsystem 1')
  SS_EastSystem2 : Subsystem
      mask Display: disp('Eastsystem 2')
  SS_NorthSystem1 : Subsystem
      mask Display: disp('Northsystem 1')
  SS_NorthSystem2 : Subsystem
      mask Display: disp('Northsystem 2')
  SS_WestSystem1 : Subsystem
      mask Display: disp('WestSystem 1')
  SS_WestSystem2 : Subsystem
      mask Display: disp('Westsystem 2')
  powergui : powerlib/powergui  SimulationMode=Discrete  SampleTime=Ts  frequency=60  Iterations=50  frequencyindice=0  Pbase=100e6  ErrMax=0.0001  UnitsV=kV  UnitsW=MW  buscounter=0  FunctionMessages=off  echomessages=off  EnableUseOfTLC=off  CurrentSourceSwitches=off  DisableSnubberDevices=off  DisableRonSwitches=off  DisableVfSwitches=off  DisplayEquations=off  AutomaticDiscreteSolvers=off  SolverType=Tustin  Interpol=off  ExternalGateDelay=off  methode=off  Ts=0  x0status=steady  SPID=off  SwTol=0  HookPort=off  NonlinearTolerance=1e-4  nMaxIteration=100  ContinueOnMaxIteration=off  RestoreLinks=warning  ResistiveCurrentMeasurement=off  Frange=[0:2:500]  Ylog=off  Xlog=on  ShowGrid=off  save=off  variable=ZData  structure=0  ZoomFFT=on  StartTime=0.0  cycles=1  DisplayStyle=1  fundamental=60  FreqAxis=off  MaxFrequency=1000  frequencyindicesteady=1  RmsSteady=2  display=off
  wires:
  SM_measurement/1(Measurements) -> SC_Console/1(Measurements)
  SM_measurement/5(ctrl_W sys2) -> SS_WestSystem2/1(ctrl_W sys 2)
  SM_measurement/6(ctrl_E sys1) -> SS_EastSystem1/1(ctrl_E sys1)
  SM_measurement/4(ctrl_W sys1) -> SS_WestSystem1/1(ctrl_W sys 1)
  SS_NorthSystem1/1(meas_N sys1) -> SM_measurement/1(meas_N sys1)
  SS_NorthSystem2/1(meas_N sys2) -> SM_measurement/2(" meas_N sys2")
  SS_EastSystem2/1(meas_E sys2) -> SM_measurement/6(measu_E sys 2)
  SS_EastSystem1/1(meas_E sys1) -> SM_measurement/5(measu_E sys 1)
  SS_WestSystem1/1(meas_W sys1) -> SM_measurement/3("meas_W sys 1  ")
  SS_WestSystem2/1(meas_W sys2) -> SM_measurement/4(" meas_W sys 2  ")
  SM_measurement/7(ctrl_E sys2) -> SS_EastSystem2/1(ctrl_E sys2)
  SM_measurement/3(ctrl_N sys2) -> SS_NorthSystem2/1(ctrl_N sys2)
  SM_measurement/2(ctrl_N sys1) -> SS_NorthSystem1/1(ctrl_N sys1)
  connections:
  Distributed Parameters Line/LConn1 -- SS_WestSystem1/RConn1
  Distributed Parameters Line/LConn2 -- SS_WestSystem1/RConn2
  Distributed Parameters Line/LConn3 -- SS_WestSystem1/RConn3
  Distributed Parameters Line1/LConn1 -- SS_WestSystem1/RConn4
  Distributed Parameters Line1/LConn2 -- SS_WestSystem1/RConn5
  Distributed Parameters Line1/LConn3 -- SS_WestSystem1/RConn6
  Distributed Parameters Line6/LConn2 -- SS_EastSystem1/LConn2
  Distributed Parameters Line6/LConn1 -- SS_EastSystem1/LConn1
  Distributed Parameters Line6/LConn3 -- SS_EastSystem1/LConn3
  SS_EastSystem1/RConn1 -- Distributed Parameters Line4/RConn1
  SS_EastSystem1/RConn2 -- Distributed Parameters Line4/RConn2
  SS_EastSystem1/RConn3 -- Distributed Parameters Line4/RConn3
  SS_EastSystem1/RConn4 -- Distributed Parameters Line5/RConn1
  SS_EastSystem1/RConn5 -- Distributed Parameters Line5/RConn2
  SS_EastSystem1/RConn6 -- Distributed Parameters Line5/RConn3
  Distributed Parameters Line/RConn1 -- SS_NorthSystem2/LConn1
  Distributed Parameters Line/RConn2 -- SS_NorthSystem2/LConn2
  Distributed Parameters Line/RConn3 -- SS_NorthSystem2/LConn3
  Distributed Parameters Line1/RConn1 -- SS_NorthSystem2/LConn4
  Distributed Parameters Line1/RConn2 -- SS_NorthSystem2/LConn5
  Distributed Parameters Line1/RConn3 -- SS_NorthSystem2/LConn6
  SS_WestSystem1/LConn1 -- Distributed Parameters Line5/LConn1
  Distributed Parameters Line5/LConn2 -- SS_WestSystem1/LConn2
  SS_WestSystem1/LConn3 -- Distributed Parameters Line5/LConn3
  Distributed Parameters Line6/RConn1 -- SS_NorthSystem2/LConn7
  Distributed Parameters Line6/RConn2 -- SS_NorthSystem2/LConn8
  Distributed Parameters Line6/RConn3 -- SS_NorthSystem2/LConn9
  Distributed Parameters Line9/RConn2 -- SS_NorthSystem1/LConn2
  Distributed Parameters Line9/LConn2 -- SS_NorthSystem2/RConn2
  Distributed Parameters Line10/RConn2 -- SS_NorthSystem1/LConn5
  Distributed Parameters Line10/LConn2 -- SS_NorthSystem2/RConn5
  Distributed Parameters Line10/RConn3 -- SS_NorthSystem1/LConn6
  Distributed Parameters Line10/RConn1 -- SS_NorthSystem1/LConn4
  Distributed Parameters Line9/RConn3 -- SS_NorthSystem1/LConn3
  Distributed Parameters Line9/RConn1 -- SS_NorthSystem1/LConn1
  Distributed Parameters Line9/LConn1 -- SS_NorthSystem2/RConn1
  Distributed Parameters Line9/LConn3 -- SS_NorthSystem2/RConn3
  SS_EastSystem1/LConn7 -- Distributed Parameters Line8/LConn1
  Distributed Parameters Line8/LConn2 -- SS_EastSystem1/LConn8
  SS_EastSystem1/LConn9 -- Distributed Parameters Line8/LConn3
  SS_EastSystem2/LConn3 -- Distributed Parameters Line8/RConn3
  Distributed Parameters Line8/RConn2 -- SS_EastSystem2/LConn2
  SS_EastSystem2/LConn1 -- Distributed Parameters Line8/RConn1
  SS_EastSystem1/LConn4 -- Distributed Parameters Line7/LConn1
  SS_EastSystem1/LConn5 -- Distributed Parameters Line7/LConn2
  SS_EastSystem1/LConn6 -- Distributed Parameters Line7/LConn3
  SS_EastSystem2/LConn4 -- Distributed Parameters Line7/RConn1
  SS_EastSystem2/LConn5 -- Distributed Parameters Line7/RConn2
  SS_EastSystem2/LConn6 -- Distributed Parameters Line7/RConn3
  SS_WestSystem2/RConn1 -- Distributed Parameters Line4/LConn1
  SS_WestSystem2/RConn2 -- Distributed Parameters Line4/LConn2
  SS_WestSystem2/RConn3 -- Distributed Parameters Line4/LConn3
  SS_WestSystem1/RConn7 -- Distributed Parameters Line2/LConn1
  Distributed Parameters Line2/LConn2 -- SS_WestSystem1/RConn8
  SS_WestSystem1/RConn9 -- Distributed Parameters Line2/LConn3
  SS_WestSystem2/LConn1 -- Distributed Parameters Line2/RConn1
  Distributed Parameters Line2/RConn2 -- SS_WestSystem2/LConn2
  SS_WestSystem2/LConn3 -- Distributed Parameters Line2/RConn3
  SS_WestSystem2/LConn4 -- Distributed Parameters Line3/RConn1
  SS_WestSystem2/LConn5 -- Distributed Parameters Line3/RConn2
  SS_WestSystem2/LConn6 -- Distributed Parameters Line3/RConn3
  Distributed Parameters Line3/LConn1 -- SS_WestSystem1/LConn4
  SS_WestSystem1/LConn5 -- Distributed Parameters Line3/LConn2
  SS_WestSystem1/LConn6 -- Distributed Parameters Line3/LConn3
  Distributed Parameters Line10/LConn1 -- SS_NorthSystem2/RConn4
  Distributed Parameters Line10/LConn3 -- SS_NorthSystem2/RConn6

== system model_FS_PSH_IEEE39/Model Initialization ==

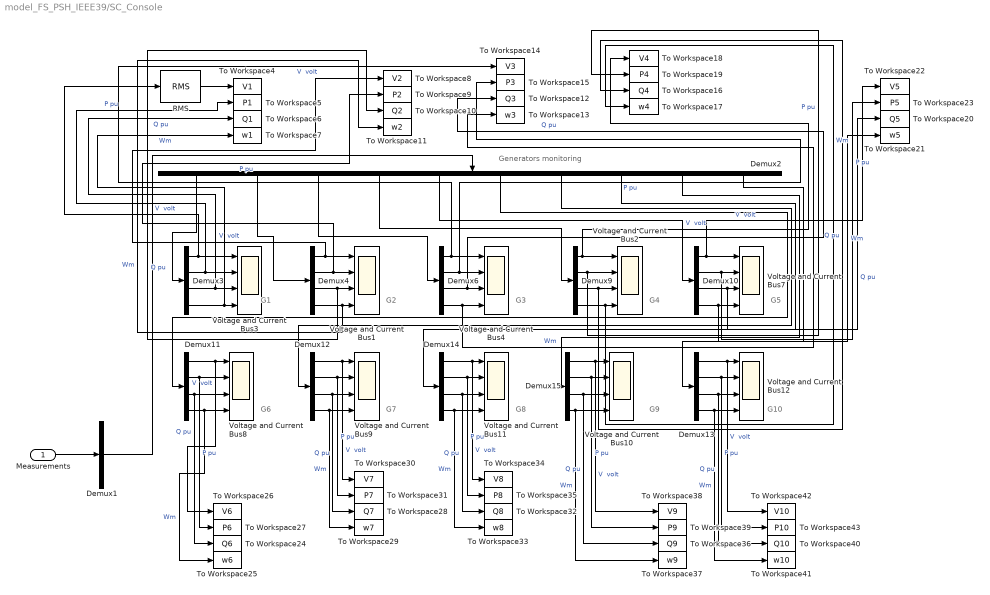
== system model_FS_PSH_IEEE39/SC_Console ==
  note: G10
  note: G9
  note: G8
  note: G7
  note: G6
  note: G5
  note: G4
  note: G3
  note: G2
  note: G1
  note: Generators monitoring
  Measurements : Inport
  Demux1 : Demux  Outputs=[60 ]
  Demux{3..4,6,9..15} (10 alike) : Demux  Outputs=[3 1 1 1]
  Demux2 : Demux  Outputs=[6 6 6 6 6 6 6 6 6 6]
  RMS : powerlib_meascontrol/Measurements/RMS  TrueRMS=on  Freq=60  RMSInit=120  Ts=0
  To Workspace10 : ToWorkspace  VariableName=Q2  SaveFormat=Timeseries  SampleTime=-1
  To Workspace11 : ToWorkspace  VariableName=w2  SaveFormat=Timeseries  SampleTime=-1
  To Workspace12 : ToWorkspace  VariableName=Q3  SaveFormat=Timeseries  SampleTime=-1
  To Workspace13 : ToWorkspace  VariableName=w3  SaveFormat=Timeseries  SampleTime=-1
  To Workspace14 : ToWorkspace  VariableName=V3  SaveFormat=Timeseries  SampleTime=-1
  To Workspace15 : ToWorkspace  VariableName=P3  SaveFormat=Timeseries  SampleTime=-1
  To Workspace16 : ToWorkspace  VariableName=Q4  SaveFormat=Timeseries  SampleTime=-1
  To Workspace17 : ToWorkspace  VariableName=w4  SaveFormat=Timeseries  SampleTime=-1
  To Workspace18 : ToWorkspace  VariableName=V4  SaveFormat=Timeseries  SampleTime=-1
  To Workspace19 : ToWorkspace  VariableName=P4  SaveFormat=Timeseries  SampleTime=-1
  To Workspace20 : ToWorkspace  VariableName=Q5  SaveFormat=Timeseries  SampleTime=-1
  To Workspace21 : ToWorkspace  VariableName=w5  SaveFormat=Timeseries  SampleTime=-1
  To Workspace22 : ToWorkspace  VariableName=V5  SaveFormat=Timeseries  SampleTime=-1
  To Workspace23 : ToWorkspace  VariableName=P5  SaveFormat=Timeseries  SampleTime=-1
  To Workspace24 : ToWorkspace  VariableName=Q6  SaveFormat=Timeseries  SampleTime=-1
  To Workspace25 : ToWorkspace  VariableName=w6  SaveFormat=Timeseries  SampleTime=-1
  To Workspace26 : ToWorkspace  VariableName=V6  SaveFormat=Timeseries  SampleTime=-1
  To Workspace27 : ToWorkspace  VariableName=P6  SaveFormat=Timeseries  SampleTime=-1
  To Workspace28 : ToWorkspace  VariableName=Q7  SaveFormat=Timeseries  SampleTime=-1
  To Workspace29 : ToWorkspace  VariableName=w7  SaveFormat=Timeseries  SampleTime=-1
  To Workspace30 : ToWorkspace  VariableName=V7  SaveFormat=Timeseries  SampleTime=-1
  To Workspace31 : ToWorkspace  VariableName=P7  SaveFormat=Timeseries  SampleTime=-1
  To Workspace32 : ToWorkspace  VariableName=Q8  SaveFormat=Timeseries  SampleTime=-1
  To Workspace33 : ToWorkspace  VariableName=w8  SaveFormat=Timeseries  SampleTime=-1
  To Workspace34 : ToWorkspace  VariableName=V8  SaveFormat=Timeseries  SampleTime=-1
  To Workspace35 : ToWorkspace  VariableName=P8  SaveFormat=Timeseries  SampleTime=-1
  To Workspace36 : ToWorkspace  VariableName=Q9  SaveFormat=Timeseries  SampleTime=-1
  To Workspace37 : ToWorkspace  VariableName=w9  SaveFormat=Timeseries  SampleTime=-1
  To Workspace38 : ToWorkspace  VariableName=V9  SaveFormat=Timeseries  SampleTime=-1
  To Workspace39 : ToWorkspace  VariableName=P9  SaveFormat=Timeseries  SampleTime=-1
  To Workspace4 : ToWorkspace  VariableName=V1  SaveFormat=Timeseries  SampleTime=-1
  To Workspace40 : ToWorkspace  VariableName=Q10  SaveFormat=Timeseries  SampleTime=-1
  To Workspace41 : ToWorkspace  VariableName=w10  SaveFormat=Timeseries  SampleTime=-1
  To Workspace42 : ToWorkspace  VariableName=V10  SaveFormat=Timeseries  SampleTime=-1
  To Workspace43 : ToWorkspace  VariableName=P10  SaveFormat=Timeseries  SampleTime=-1
  To Workspace5 : ToWorkspace  VariableName=P1  SaveFormat=Timeseries  SampleTime=-1
  To Workspace6 : ToWorkspace  VariableName=Q1  SaveFormat=Timeseries  SampleTime=-1
  To Workspace7 : ToWorkspace  VariableName=w1  SaveFormat=Timeseries  SampleTime=-1
  To Workspace8 : ToWorkspace  VariableName=V2  SaveFormat=Timeseries  SampleTime=-1
  To Workspace9 : ToWorkspace  VariableName=P2  SaveFormat=Timeseries  SampleTime=-1
  Voltage and Current Bus{1..4,7..12} (10 alike) : Scope  NumInputPorts=4
  wires:
  Demux1/1 -> Demux2/1
  Demux2/10 -> Demux13/1
  Demux2/9 -> Demux15/1
  Demux2/8 -> Demux14/1
  Demux2/7 -> Demux12/1
  Demux2/6 -> Demux11/1
  Demux2/5 -> Demux10/1
  Demux2/4 -> Demux9/1
  Demux2/3 -> Demux6/1
  Demux2/2 -> Demux4/1
  Demux2/1 -> Demux3/1
  Measurements/1 -> Demux1/1
  Demux3/1 -> Voltage and Current Bus3/1, RMS/1  "V  volt"
  Demux3/3 -> To Workspace6/1, Voltage and Current Bus3/3  "Q pu"
  Demux3/4 -> To Workspace7/1, Voltage and Current Bus3/4  "Wm"
  Demux3/2 -> To Workspace5/1, Voltage and Current Bus3/2  "P pu"
  Demux4/1 -> To Workspace8/1, Voltage and Current Bus1/1  "V  volt"
  Demux4/3 -> To Workspace10/1, Voltage and Current Bus1/3  "Q pu"
  Demux4/4 -> To Workspace11/1, Voltage and Current Bus1/4  "Wm"
  Demux4/2 -> To Workspace9/1, Voltage and Current Bus1/2  "P pu"
  Demux6/1 -> To Workspace14/1, Voltage and Current Bus4/1  "V  volt"
  Demux6/3 -> To Workspace12/1, Voltage and Current Bus4/3  "Q pu"
  Demux6/4 -> To Workspace13/1, Voltage and Current Bus4/4  "Wm"
  Demux6/2 -> To Workspace15/1, Voltage and Current Bus4/2  "P pu"
  Demux9/1 -> To Workspace18/1, Voltage and Current Bus2/1  "V  volt"
  Demux9/3 -> To Workspace16/1, Voltage and Current Bus2/3  "Q pu"
  Demux9/4 -> To Workspace17/1, Voltage and Current Bus2/4  "Wm"
  Demux9/2 -> To Workspace19/1, Voltage and Current Bus2/2  "P pu"
  Demux10/1 -> To Workspace22/1, Voltage and Current Bus7/1  "V  volt"
  Demux10/3 -> To Workspace20/1, Voltage and Current Bus7/3  "Q pu"
  Demux10/4 -> To Workspace21/1, Voltage and Current Bus7/4  "Wm"
  Demux10/2 -> To Workspace23/1, Voltage and Current Bus7/2  "P pu"
  Demux11/1 -> To Workspace26/1, Voltage and Current Bus8/1  "V  volt"
  Demux11/3 -> Voltage and Current Bus8/3, To Workspace24/1  "Q pu"
  Demux11/4 -> To Workspace25/1, Voltage and Current Bus8/4  "Wm"
  Demux11/2 -> Voltage and Current Bus8/2, To Workspace27/1  "P pu"
  Demux12/1 -> To Workspace30/1, Voltage and Current Bus9/1  "V  volt"
  Demux12/3 -> To Workspace28/1, Voltage and Current Bus9/3  "Q pu"
  Demux12/4 -> To Workspace29/1, Voltage and Current Bus9/4  "Wm"
  Demux12/2 -> To Workspace31/1, Voltage and Current Bus9/2  "P pu"
  Demux14/1 -> To Workspace34/1, Voltage and Current Bus11/1  "V  volt"
  Demux14/3 -> To Workspace32/1, Voltage and Current Bus11/3  "Q pu"
  Demux14/4 -> To Workspace33/1, Voltage and Current Bus11/4  "Wm"
  Demux14/2 -> To Workspace35/1, Voltage and Current Bus11/2  "P pu"
  Demux15/1 -> To Workspace38/1, Voltage and Current Bus10/1  "V  volt"
  Demux15/3 -> To Workspace36/1, Voltage and Current Bus10/3  "Q pu"
  Demux15/4 -> To Workspace37/1, Voltage and Current Bus10/4  "Wm"
  Demux15/2 -> To Workspace39/1, Voltage and Current Bus10/2  "P pu"
  Demux13/1 -> To Workspace42/1, Voltage and Current Bus12/1  "V  volt"
  Demux13/3 -> To Workspace40/1, Voltage and Current Bus12/3  "Q pu"
  Demux13/4 -> To Workspace41/1, Voltage and Current Bus12/4  "Wm"
  Demux13/2 -> To Workspace43/1, Voltage and Current Bus12/2  "P pu"
  RMS/1 -> To Workspace4/1

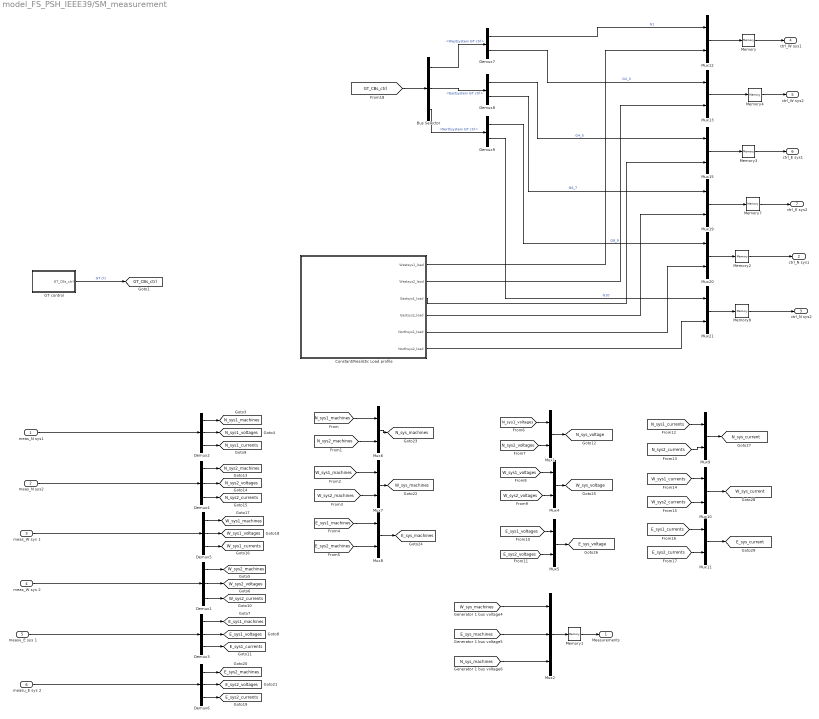
== system model_FS_PSH_IEEE39/SM_measurement ==
  meas_N sys1 : Inport
  " meas_N sys2" : Inport  Port=2
  "meas_W sys 1  " : Inport  Port=3
  " meas_W sys 2  " : Inport  Port=4
  measu_E sys 1 : Inport  Port=5
  measu_E sys 2 : Inport  Port=6
  Bus Selector : BusSelector  OutputSignals=Westsystem GT ctrl,Eastsystem GT ctrl,Northsystem GT ctrl
  Constant/Realistic Load profile : Subsystem  SystemSampleTime=20e-3  mask{Loadselect=Constant Load}
      mask init:
      | if (Loadselect == 1)
      |     mode = 0;
      | else 
      |         mode = 1; 
      | end
      mask TypeOptions Loadselect: Constant Load | Realistic Load
      mask Display: disp('Load Profile \n Constant / Realistic')
  Demux1 : Demux  Outputs=[12 18 18]
  Demux2 : Demux  Outputs=[12 12 12]
  Demux3 : Demux  Outputs=[12 15 15]
  Demux4 : Demux  Outputs=[6 18 18]
  Demux5 : Demux  Outputs=[6 15 15]
  Demux6 : Demux  Outputs=[12 12 12]
  Demux7 : Demux  Outputs=[1 2]
  Demux8 : Demux  Outputs=[2 2]
  Demux9 : Demux  Outputs=[2 1]
  GT control : Subsystem
  Memory{,1..4,7..8} (7 alike) : Memory
  Mux{1,4..13,15,19..21} (15 alike) : Mux  Inputs=2
  Mux2 : Mux  Inputs=3
  Measurements : Outport
  ctrl_N sys1 : Outport  Port=2
  ctrl_N sys2 : Outport  Port=3
  ctrl_W sys1 : Outport  Port=4
  ctrl_W sys2 : Outport  Port=5
  ctrl_E sys1 : Outport  Port=6
  ctrl_E sys2 : Outport  Port=7
  tag scope: E_sys1_currents=global, E_sys1_machines=global, E_sys1_voltages=global, E_sys2_currents=global, E_sys2_machines=global, E_sys2_voltages=global, E_sys_current=global, E_sys_machines=global, E_sys_voltage=global, GT_CBs_ctrl=global, N_sys1_currents=global, N_sys1_machines=global, N_sys1_voltages=global, N_sys2_currents=global, N_sys2_machines=global, N_sys2_voltages=global, N_sys_current=global, N_sys_machines=global, N_sys_voltage=global, W_sys1_currents=global, W_sys1_machines=global, W_sys1_voltages=global, W_sys2_currents=global, W_sys2_machines=global, W_sys2_voltages=global, W_sys_current=global, W_sys_machines=global, W_sys_voltage=global
  wires:
  Demux3/2 -> [E_sys1_voltages]
  Demux1/2 -> [W_sys2_voltages]
  Demux2/2 -> [N_sys1_voltages]
  Memory1/1 -> Measurements/1
  [N_sys_machines] -> Mux2/3
  [E_sys_machines] -> Mux2/2
  [W_sys_machines] -> Mux2/1
  Demux3/1 -> [E_sys1_machines]
  Demux1/1 -> [W_sys2_machines]
  Mux2/1 -> Memory1/1
  meas_N sys1/1 -> Demux2/1
  Demux2/1 -> [N_sys1_machines]
  Demux2/3 -> [N_sys1_currents]
  Demux1/3 -> [W_sys2_currents]
  Demux3/3 -> [E_sys1_currents]
  GT control/1(GT_CBs_ctrl) -> [GT_CBs_ctrl]  "GT ctr"
  Demux4/2 -> [N_sys2_voltages]
  Demux4/1 -> [N_sys2_machines]
  Demux4/3 -> [N_sys2_currents]
  " meas_N sys2"/1 -> Demux4/1
  " meas_W sys 2  "/1 -> Demux1/1
  Demux5/2 -> [W_sys1_voltages]
  Demux5/1 -> [W_sys1_machines]
  Demux5/3 -> [W_sys1_currents]
  "meas_W sys 1  "/1 -> Demux5/1
  measu_E sys 1/1 -> Demux3/1
  Demux6/2 -> [E_sys2_voltages]
  Demux6/1 -> [E_sys2_machines]
  Demux6/3 -> [E_sys2_currents]
  measu_E sys 2/1 -> Demux6/1
  [N_sys2_machines] -> Mux6/2
  [N_sys1_machines] -> Mux6/1
  Mux6/1 -> [N_sys_machines]
  [W_sys1_machines] -> Mux7/1
  [W_sys2_machines] -> Mux7/2
  Mux7/1 -> [W_sys_machines]
  [E_sys1_machines] -> Mux8/1
  [E_sys2_machines] -> Mux8/2
  Mux8/1 -> [E_sys_machines]
  [N_sys1_voltages] -> Mux1/1
  [N_sys2_voltages] -> Mux1/2
  [W_sys1_voltages] -> Mux4/1
  [W_sys2_voltages] -> Mux4/2
  [E_sys1_voltages] -> Mux5/1
  [E_sys2_voltages] -> Mux5/2
  Mux1/1 -> [N_sys_voltage]
  Mux4/1 -> [W_sys_voltage]
  Mux5/1 -> [E_sys_voltage]
  [N_sys1_currents] -> Mux9/1
  [N_sys2_currents] -> Mux9/2
  [W_sys1_currents] -> Mux10/1
  [W_sys2_currents] -> Mux10/2
  [E_sys1_currents] -> Mux11/1
  [E_sys2_currents] -> Mux11/2
  Mux9/1 -> [N_sys_current]
  Mux10/1 -> [W_sys_current]
  Mux11/1 -> [E_sys_current]
  Memory2/1 -> ctrl_N sys1/1
  Memory3/1 -> ctrl_E sys1/1
  Memory/1 -> ctrl_W sys1/1
  Constant/Realistic Load profile/1(Westsys1_load) -> Mux12/2
  Constant/Realistic Load profile/2(Westsys2_laod) -> Mux13/2
  Memory4/1 -> ctrl_W sys2/1
  Constant/Realistic Load profile/3(Eastsys1_load) -> Mux15/2
  Constant/Realistic Load profile/4(Eastsys2_load) -> Mux19/2
  Memory7/1 -> ctrl_E sys2/1
  Constant/Realistic Load profile/5(Northsys1_load) -> Mux20/2
  Constant/Realistic Load profile/6(Northsys2_load) -> Mux21/2
  Memory8/1 -> ctrl_N sys2/1
  Mux20/1 -> Memory2/1
  [GT_CBs_ctrl] -> Bus Selector/1
  Bus Selector/2 -> Demux8/1  "<Eastsystem GT ctrl>"
  Bus Selector/1 -> Demux7/1  "<Westsystem GT ctrl>"
  Bus Selector/3 -> Demux9/1  "<Northsystem GT ctrl>"
  Demux7/1 -> Mux12/1  "G1"
  Mux12/1 -> Memory/1
  Demux7/2 -> Mux13/1  "G2_3"
  Mux13/1 -> Memory4/1
  Demux8/1 -> Mux15/1  "G4_5"
  Demux8/2 -> Mux19/1  "G6_7"
  Mux15/1 -> Memory3/1
  Mux19/1 -> Memory7/1
  Demux9/1 -> Mux20/1  "G8_9"
  Demux9/2 -> Mux21/1  "G10"
  Mux21/1 -> Memory8/1
